simulink library "Batteries"  (R2023b)
settings: Solver=VariableStepAuto  StartTime=0.0  StopTime=10.0  RelTol=1e-3
undefined symbols (not defined in the file or in its folder): battery_builder_rtmsupport, gcbh
libraries: Batteries_lib x8
(part 1 of 4)
settings Model: Creator=maxju  LastModifiedBy=maxju

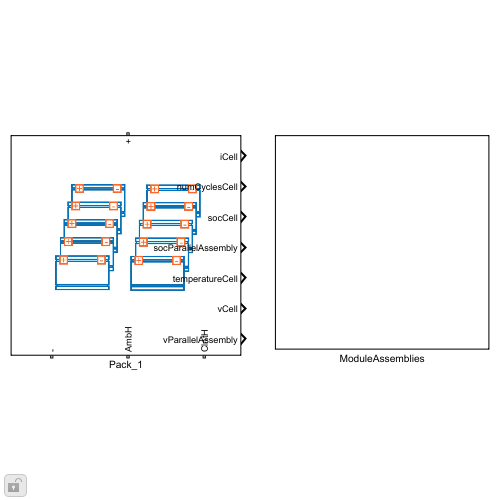
[thumbnail: Simulink's stored preview of the top-level diagram]
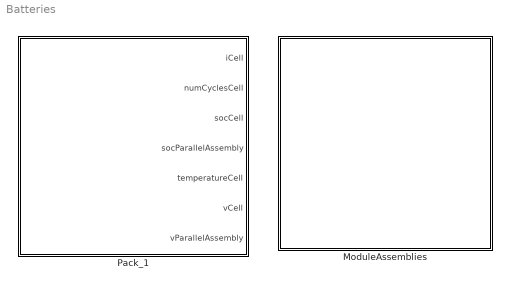
== system Batteries ==
  ModuleAssemblies : Subsystem
  Pack_1 : Subsystem  LoadFcn=battery_builder_rtmsupport('loadfcn',gcbh);
      settings: CopyFcn=battery_builder_rtmsupport('copyfcn',gcbh);  PreCopyFcn=battery_builder_rtmsupport('precopyfcn',gcbh);  PreDeleteFcn=battery_builder_rtmsupport('predeletefcn',gcbh);  PortSchema="{\"entries\":[{\"content\":{\"sides\":[{\"content\":{\"connectorIds\":[\"LConn1\"]},\"type\":\"ConnectorPlacement.EquallySpacedRectSide\",\"uuid\":\"3208743a-a519-41a1-8ebe-6eed9670d19c\"},{\"content\":{\"connectorIds\":[\"RConn1\",\"RConn2\",\"RConn3\"],\"side\":\"RIGHT\"},\"type\":\"ConnectorPlacement.EquallySpacedRectSide\",\"uuid\":\"e7c9afcf-26e4-4003-a175-67ec4307a0b6\"},{\"content\":{\"side\":\"TOP\"},\"type\":\"ConnectorPlacement.EquallySpacedRectSide\",\"uuid\":\"e113849d-7e09-4ac7-ac0d-e10ce5f1c420\"},{\"content\":{\"connectorIds\":[\"Out1\",\"Out2\",\"Out3\",\"Out4\",\"Out5\",\"Out6\",\"Out7\"],\"side\":\"BOTTOM\"},\"type\":\"ConnectorPlacement.EquallySpacedRectSide\",\"uuid\":\"7e3d0ba5-349a-464e-b9e7-0ee2ee84a6c1\"}]},\"type\":\"ConnectorPlacement.EquallySpacedConnector\",\"uuid\":\"9e673d86-8bc3-4af2-b5cc-e8b6c563b87a\"}],\"packageUris\":[\"http://schema.mathworks.com/mf0/Connector/R2020b\"],\"version\":\"1.0\"}"
      mask Display: image('$imagefile')

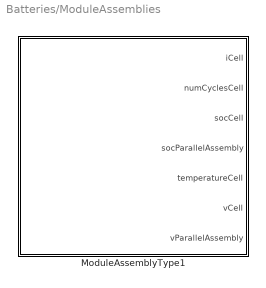
== system Batteries/ModuleAssemblies ==
  ModuleAssemblyType1 : Subsystem  LoadFcn=battery_builder_rtmsupport('loadfcn',gcbh);
      settings: CopyFcn=battery_builder_rtmsupport('copyfcn',gcbh);  PreCopyFcn=battery_builder_rtmsupport('precopyfcn',gcbh);  PreDeleteFcn=battery_builder_rtmsupport('predeletefcn',gcbh);  PortSchema="{\"entries\":[{\"content\":{\"sides\":[{\"content\":{\"connectorIds\":[\"LConn1\"]},\"type\":\"ConnectorPlacement.EquallySpacedRectSide\",\"uuid\":\"3208743a-a519-41a1-8ebe-6eed9670d19c\"},{\"content\":{\"connectorIds\":[\"RConn1\",\"RConn2\",\"RConn3\"],\"side\":\"RIGHT\"},\"type\":\"ConnectorPlacement.EquallySpacedRectSide\",\"uuid\":\"e7c9afcf-26e4-4003-a175-67ec4307a0b6\"},{\"content\":{\"side\":\"TOP\"},\"type\":\"ConnectorPlacement.EquallySpacedRectSide\",\"uuid\":\"e113849d-7e09-4ac7-ac0d-e10ce5f1c420\"},{\"content\":{\"connectorIds\":[\"Out1\",\"Out2\",\"Out3\",\"Out4\",\"Out5\",\"Out6\",\"Out7\"],\"side\":\"BOTTOM\"},\"type\":\"ConnectorPlacement.EquallySpacedRectSide\",\"uuid\":\"c73d48af-17c4-4fef-bb81-c5ffd3e9339e\"}]},\"type\":\"ConnectorPlacement.EquallySpacedConnector\",\"uuid\":\"9e673d86-8bc3-4af2-b5cc-e8b6c563b87a\"}],\"packageUris\":[\"http://schema.mathworks.com/mf0/Connector/R2020b\"],\"version\":\"1.0\"}"
      mask Display: image('$imagefile')

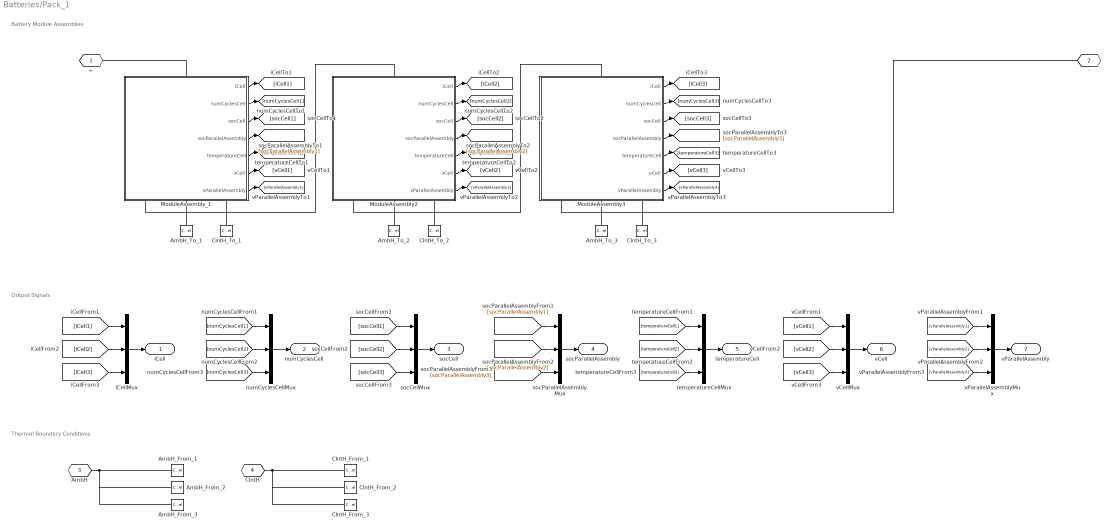
== system Batteries/Pack_1 ==
  note: Battery Module Assemblies
  note: Output Signals
  note: Thermal Boundary Conditions
  AmbH_From_1 : ConnectionLabel  Label=ambH_1
  AmbH_From_2 : ConnectionLabel  Label=ambH_2
  AmbH_From_3 : ConnectionLabel  Label=ambH_3
  AmbH_To_1 : ConnectionLabel  Label=ambH_1
  AmbH_To_2 : ConnectionLabel  Label=ambH_2
  AmbH_To_3 : ConnectionLabel  Label=ambH_3
  ClntH_From_1 : ConnectionLabel  Label=clntH_1
  ClntH_From_2 : ConnectionLabel  Label=clntH_2
  ClntH_From_3 : ConnectionLabel  Label=clntH_3
  ClntH_To_1 : ConnectionLabel  Label=clntH_1
  ClntH_To_2 : ConnectionLabel  Label=clntH_2
  ClntH_To_3 : ConnectionLabel  Label=clntH_3
  ModuleAssembly2 : Subsystem  LoadFcn=battery_builder_rtmsupport('loadfcn',gcbh);
      settings: CopyFcn=battery_builder_rtmsupport('copyfcn',gcbh);  PreCopyFcn=battery_builder_rtmsupport('precopyfcn',gcbh);  PreDeleteFcn=battery_builder_rtmsupport('predeletefcn',gcbh);  PortSchema="{\"entries\":[{\"content\":{\"sides\":[{\"content\":{\"connectorIds\":[\"LConn1\"]},\"type\":\"ConnectorPlacement.EquallySpacedRectSide\",\"uuid\":\"3208743a-a519-41a1-8ebe-6eed9670d19c\"},{\"content\":{\"connectorIds\":[\"RConn1\",\"RConn2\",\"RConn3\"],\"side\":\"RIGHT\"},\"type\":\"ConnectorPlacement.EquallySpacedRectSide\",\"uuid\":\"e7c9afcf-26e4-4003-a175-67ec4307a0b6\"},{\"content\":{\"side\":\"TOP\"},\"type\":\"ConnectorPlacement.EquallySpacedRectSide\",\"uuid\":\"e113849d-7e09-4ac7-ac0d-e10ce5f1c420\"},{\"content\":{\"connectorIds\":[\"Out1\",\"Out2\",\"Out3\",\"Out4\",\"Out5\",\"Out6\",\"Out7\"],\"side\":\"BOTTOM\"},\"type\":\"ConnectorPlacement.EquallySpacedRectSide\",\"uuid\":\"c73d48af-17c4-4fef-bb81-c5ffd3e9339e\"}]},\"type\":\"ConnectorPlacement.EquallySpacedConnector\",\"uuid\":\"9e673d86-8bc3-4af2-b5cc-e8b6c563b87a\"}],\"packageUris\":[\"http://schema.mathworks.com/mf0/Connector/R2020b\"],\"version\":\"1.0\"}"
      mask Display: image('$imagefile')
  ModuleAssembly3 : Subsystem  LoadFcn=battery_builder_rtmsupport('loadfcn',gcbh);
      settings: CopyFcn=battery_builder_rtmsupport('copyfcn',gcbh);  PreCopyFcn=battery_builder_rtmsupport('precopyfcn',gcbh);  PreDeleteFcn=battery_builder_rtmsupport('predeletefcn',gcbh);  PortSchema="{\"entries\":[{\"content\":{\"sides\":[{\"content\":{\"connectorIds\":[\"LConn1\"]},\"type\":\"ConnectorPlacement.EquallySpacedRectSide\",\"uuid\":\"3208743a-a519-41a1-8ebe-6eed9670d19c\"},{\"content\":{\"connectorIds\":[\"RConn1\",\"RConn2\",\"RConn3\"],\"side\":\"RIGHT\"},\"type\":\"ConnectorPlacement.EquallySpacedRectSide\",\"uuid\":\"e7c9afcf-26e4-4003-a175-67ec4307a0b6\"},{\"content\":{\"side\":\"TOP\"},\"type\":\"ConnectorPlacement.EquallySpacedRectSide\",\"uuid\":\"e113849d-7e09-4ac7-ac0d-e10ce5f1c420\"},{\"content\":{\"connectorIds\":[\"Out1\",\"Out2\",\"Out3\",\"Out4\",\"Out5\",\"Out6\",\"Out7\"],\"side\":\"BOTTOM\"},\"type\":\"ConnectorPlacement.EquallySpacedRectSide\",\"uuid\":\"c73d48af-17c4-4fef-bb81-c5ffd3e9339e\"}]},\"type\":\"ConnectorPlacement.EquallySpacedConnector\",\"uuid\":\"9e673d86-8bc3-4af2-b5cc-e8b6c563b87a\"}],\"packageUris\":[\"http://schema.mathworks.com/mf0/Connector/R2020b\"],\"version\":\"1.0\"}"
      mask Display: image('$imagefile')
  ModuleAssembly_1 : Subsystem  LoadFcn=battery_builder_rtmsupport('loadfcn',gcbh);
      settings: CopyFcn=battery_builder_rtmsupport('copyfcn',gcbh);  PreCopyFcn=battery_builder_rtmsupport('precopyfcn',gcbh);  PreDeleteFcn=battery_builder_rtmsupport('predeletefcn',gcbh);  PortSchema="{\"entries\":[{\"content\":{\"sides\":[{\"content\":{\"connectorIds\":[\"LConn1\"]},\"type\":\"ConnectorPlacement.EquallySpacedRectSide\",\"uuid\":\"3208743a-a519-41a1-8ebe-6eed9670d19c\"},{\"content\":{\"connectorIds\":[\"RConn1\",\"RConn2\",\"RConn3\"],\"side\":\"RIGHT\"},\"type\":\"ConnectorPlacement.EquallySpacedRectSide\",\"uuid\":\"e7c9afcf-26e4-4003-a175-67ec4307a0b6\"},{\"content\":{\"side\":\"TOP\"},\"type\":\"ConnectorPlacement.EquallySpacedRectSide\",\"uuid\":\"e113849d-7e09-4ac7-ac0d-e10ce5f1c420\"},{\"content\":{\"connectorIds\":[\"Out1\",\"Out2\",\"Out3\",\"Out4\",\"Out5\",\"Out6\",\"Out7\"],\"side\":\"BOTTOM\"},\"type\":\"ConnectorPlacement.EquallySpacedRectSide\",\"uuid\":\"c73d48af-17c4-4fef-bb81-c5ffd3e9339e\"}]},\"type\":\"ConnectorPlacement.EquallySpacedConnector\",\"uuid\":\"9e673d86-8bc3-4af2-b5cc-e8b6c563b87a\"}],\"packageUris\":[\"http://schema.mathworks.com/mf0/Connector/R2020b\"],\"version\":\"1.0\"}"
      mask Display: image('$imagefile')
  iCellMux : Mux  Inputs=3
  numCyclesCellMux : Mux  Inputs=3
  socCellMux : Mux  Inputs=3
  socParallelAssemblyMux : Mux  Inputs=3
  temperatureCellMux : Mux  Inputs=3
  vCellMux : Mux  Inputs=3
  vParallelAssemblyMux : Mux  Inputs=3
  + : PMIOPort  Side=Left
  - : PMIOPort  Port=2  Side=Right
  AmbH : PMIOPort  Port=3  Side=Right  ConnectionType=Connection: foundation.thermal.thermal
  ClntH : PMIOPort  Port=4  Side=Right  ConnectionType=Connection: foundation.thermal.thermal
  iCell : Outport
  numCyclesCell : Outport  Port=2
  socCell : Outport  Port=3
  socParallelAssembly : Outport  Port=4
  temperatureCell : Outport  Port=5
  vCell : Outport  Port=6
  vParallelAssembly : Outport  Port=7
  wires:
  ModuleAssembly_1/1(iCell) -> [iCell1]
  iCellMux/1 -> iCell/1
  [iCell1] -> iCellMux/1
  ModuleAssembly_1/2(numCyclesCell) -> [numCyclesCell1]
  numCyclesCellMux/1 -> numCyclesCell/1
  [numCyclesCell1] -> numCyclesCellMux/1
  ModuleAssembly_1/3(socCell) -> [socCell1]
  socCellMux/1 -> socCell/1
  [socCell1] -> socCellMux/1
  ModuleAssembly_1/4(socParallelAssembly) -> [socParallelAssembly1]
  socParallelAssemblyMux/1 -> socParallelAssembly/1
  [socParallelAssembly1] -> socParallelAssemblyMux/1
  ModuleAssembly_1/5(temperatureCell) -> [temperatureCell1]
  temperatureCellMux/1 -> temperatureCell/1
  [temperatureCell1] -> temperatureCellMux/1
  ModuleAssembly_1/6(vCell) -> [vCell1]
  vCellMux/1 -> vCell/1
  [vCell1] -> vCellMux/1
  ModuleAssembly_1/7(vParallelAssembly) -> [vParallelAssembly1]
  vParallelAssemblyMux/1 -> vParallelAssembly/1
  [vParallelAssembly1] -> vParallelAssemblyMux/1
  ModuleAssembly2/1(iCell) -> [iCell2]
  [iCell2] -> iCellMux/2
  ModuleAssembly2/2(numCyclesCell) -> [numCyclesCell2]
  [numCyclesCell2] -> numCyclesCellMux/2
  ModuleAssembly2/3(socCell) -> [socCell2]
  [socCell2] -> socCellMux/2
  ModuleAssembly2/4(socParallelAssembly) -> [socParallelAssembly2]
  [socParallelAssembly2] -> socParallelAssemblyMux/2
  ModuleAssembly2/5(temperatureCell) -> [temperatureCell2]
  [temperatureCell2] -> temperatureCellMux/2
  ModuleAssembly2/6(vCell) -> [vCell2]
  [vCell2] -> vCellMux/2
  ModuleAssembly2/7(vParallelAssembly) -> [vParallelAssembly2]
  [vParallelAssembly2] -> vParallelAssemblyMux/2
  ModuleAssembly3/1(iCell) -> [iCell3]
  [iCell3] -> iCellMux/3
  ModuleAssembly3/2(numCyclesCell) -> [numCyclesCell3]
  [numCyclesCell3] -> numCyclesCellMux/3
  ModuleAssembly3/3(socCell) -> [socCell3]
  [socCell3] -> socCellMux/3
  ModuleAssembly3/4(socParallelAssembly) -> [socParallelAssembly3]
  [socParallelAssembly3] -> socParallelAssemblyMux/3
  ModuleAssembly3/5(temperatureCell) -> [temperatureCell3]
  [temperatureCell3] -> temperatureCellMux/3
  ModuleAssembly3/6(vCell) -> [vCell3]
  [vCell3] -> vCellMux/3
  ModuleAssembly3/7(vParallelAssembly) -> [vParallelAssembly3]
  [vParallelAssembly3] -> vParallelAssemblyMux/3
  connections:
  ModuleAssembly2/LConn1 -- ModuleAssembly_1/RConn1
  ModuleAssembly3/LConn1 -- ModuleAssembly2/RConn1
  ModuleAssembly_1/LConn1 -- +/RConn1
  ModuleAssembly3/RConn1 -- -/RConn1
  AmbH_To_1/LConn1 -- ModuleAssembly_1/RConn2
  AmbH_From_1/LConn1 -- AmbH_From_2/LConn1 -- AmbH/RConn1 -- AmbH_From_3/LConn1
  AmbH_To_2/LConn1 -- ModuleAssembly2/RConn2
  AmbH_To_3/LConn1 -- ModuleAssembly3/RConn2
  ClntH_To_1/LConn1 -- ModuleAssembly_1/RConn3
  ClntH_From_1/LConn1 -- ClntH_From_2/LConn1 -- ClntH/RConn1 -- ClntH_From_3/LConn1
  ClntH_To_2/LConn1 -- ModuleAssembly2/RConn3
  ClntH_To_3/LConn1 -- ModuleAssembly3/RConn3

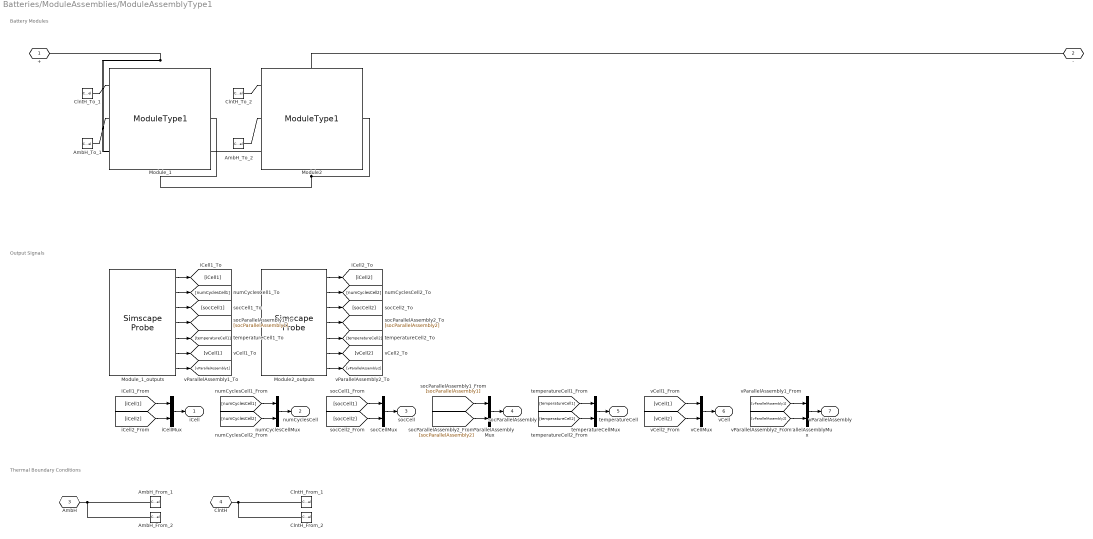
== system Batteries/ModuleAssemblies/ModuleAssemblyType1 ==
  note: Battery Modules
  note: Output Signals
  note: Thermal Boundary Conditions
  AmbH_From_1 : ConnectionLabel  Label=ambH_1
  AmbH_From_2 : ConnectionLabel  Label=ambH_2
  AmbH_To_1 : ConnectionLabel  Label=ambH_1
  AmbH_To_2 : ConnectionLabel  Label=ambH_2
  ClntH_From_1 : ConnectionLabel  Label=clntH_1
  ClntH_From_2 : ConnectionLabel  Label=clntH_2
  ClntH_To_1 : ConnectionLabel  Label=clntH_1
  ClntH_To_2 : ConnectionLabel  Label=clntH_2
  Module2 : Batteries_lib/Modules/ModuleType1  SOC_vecCell=[0, .01, .02, .03, .04, .05, .06, .07, .08, .09, .1, .11, .12, .13, .14, .15, .16, .17, .18, .19, .2, .21, .22, .23, .24, .25, .26, .27, .28, .29, .3, .31, .32, .33, .34, .35, .36, .37, .38, .39, .4, .41, .42, .43, .44, .45, .46, .47, .48, .49, .5, .51, .52, .53, .54, .55, .56, .57, .58, .59, .6, .61, .62, .63, .64, .65, .66, .67, .68, .69, .7, .71, .72, .73, .74, .75, .76, .77, .78, .79, .8, .81, .82, .83, .84, .85, .86, .87, .88, .89, .9, .91, .92, .93, .94, .95, .96, .97, .98, .99, 1]  T_vecCell=[-10, 0, 25, 40, 60] degC  V0_matCell=[2.90003, 2.90003, 2.90003, 2.90003, 2.90003; 2.94341, 2.94341, 2.94341, 2.94341, 2.94341; 2.98679, 2.98679, 2.98679, 2.98679, 2.98679; 3.04987, 3.04987, 3.04987, 3.04987, 3.04987; 3.09433, 3.09433, 3.09433, 3.09433, 3.09433; 3.12791, 3.12791, 3.12791, 3.12791, 3.12791; 3.16031, 3.16031, 3.16031, 3.16031, 3.16031; 3.20369, 3.20369, 3.20369, 3.20369, 3.20369; 3.23862, 3.23862, 3.23862, 3.23862, 3.23862; 3.26689, 3.26689, 3.26689, 3.26689, 3.26689; 3.29115, 3.29115, 3.29115, 3.29115, 3.29115; 3.31383, 3.31383, 3.31383, 3.31383, 3.31383; 3.33202, 3.33202, 3.33202, 3.33202, 3.33202; 3.35112, 3.35112, 3.35112, 3.35112, 3.35112; 3.36833, 3.36833, 3.36833, 3.36833, 3.36833; 3.38413, 3.38413, 3.38413, 3.38413, 3.38413; 3.39973, 3.39973, 3.39973, 3.39973, 3.39973; 3.41137, 3.41137, 3.41137, 3.41137, 3.41137; 3.42149, 3.42149, 3.42149, 3.42149, 3.42149; 3.43136, 3.43136, 3.43136, 3.43136, 3.43136; 3.44073, 3.44073, 3.44073, 3.44073, 3.44073; 3.45027, 3.45027, 3.45027, 3.45027, 3.45027; 3.46068, 3.46068, 3.46068, 3.46068, 3.46068; 3.47113, 3.47113, 3.47113, 3.47113, 3.47113; 3.47814, 3.47814, 3.47814, 3.47814, 3.47814; 3.48494, 3.48494, 3.48494, 3.48494, 3.48494; 3.49199, 3.49199, 3.49199, 3.49199, 3.49199; 3.49905, 3.49905, 3.49905, 3.49905, 3.49905; 3.50562, 3.50562, 3.50562, 3.50562, 3.50562; 3.51187, 3.51187, 3.51187, 3.51187, 3.51187; 3.51861, 3.51861, 3.51861, 3.51861, 3.51861; 3.52535, 3.52535, 3.52535, 3.52535, 3.52535; 3.53209, 3.53209, 3.53209, 3.53209, 3.53209; 3.53818, 3.53818, 3.53818, 3.53818, 3.53818; 3.54353, 3.54353, 3.54353, 3.54353, 3.54353; 3.54849, 3.54849, 3.54849, 3.54849, 3.54849; 3.55353, 3.55353, 3.55353, 3.55353, 3.55353; 3.55855, 3.55855, 3.55855, 3.55855, 3.55855; 3.56357, 3.56357, 3.56357, 3.56357, 3.56357; 3.56831, 3.56831, 3.56831, 3.56831, 3.56831; 3.57308, 3.57308, 3.57308, 3.57308, 3.57308; 3.57787, 3.57787, 3.57787, 3.57787, 3.57787; 3.58264, 3.58264, 3.58264, 3.58264, 3.58264; 3.58755, 3.58755, 3.58755, 3.58755, 3.58755; 3.5925, 3.5925, 3.5925, 3.5925, 3.5925; 3.5985, 3.5985, 3.5985, 3.5985, 3.5985; 3.60496, 3.60496, 3.60496, 3.60496, 3.60496; 3.61149, 3.61149, 3.61149, 3.61149, 3.61149; 3.61805, 3.61805, 3.61805, 3.61805, 3.61805; 3.6246, 3.6246, 3.6246, 3.6246, 3.6246; 3.63116, 3.63116, 3.63116, 3.63116, 3.63116; 3.63855, 3.63855, 3.63855, 3.63855, 3.63855; 3.64609, 3.64609, 3.64609, 3.64609, 3.64609; 3.65336, 3.65336, 3.65336, 3.65336, 3.65336; 3.66064, 3.66064, 3.66064, 3.66064, 3.66064; 3.66791, 3.66791, 3.66791, 3.66791, 3.66791; 3.67613, 3.67613, 3.67613, 3.67613, 3.67613; 3.68522, 3.68522, 3.68522, 3.68522, 3.68522; 3.69443, 3.69443, 3.69443, 3.69443, 3.69443; 3.70367, 3.70367, 3.70367, 3.70367, 3.70367; 3.713, 3.713, 3.713, 3.713, 3.713; 3.72241, 3.72241, 3.72241, 3.72241, 3.72241; 3.73154, 3.73154, 3.73154, 3.73154, 3.73154; 3.74037, 3.74037, 3.74037, 3.74037, 3.74037; 3.7492, 3.7492, 3.7492, 3.7492, 3.7492; 3.75786, 3.75786, 3.75786, 3.75786, 3.75786; 3.76617, 3.76617, 3.76617, 3.76617, 3.76617; 3.77556, 3.77556, 3.77556, 3.77556, 3.77556; 3.78485, 3.78485, 3.78485, 3.78485, 3.78485; 3.79413, 3.79413, 3.79413, 3.79413, 3.79413; 3.8034, 3.8034, 3.8034, 3.8034, 3.8034; 3.81149, 3.81149, 3.81149, 3.81149, 3.81149; 3.81977, 3.81977, 3.81977, 3.81977, 3.81977; 3.82804, 3.82804, 3.82804, 3.82804, 3.82804; 3.83631, 3.83631, 3.83631, 3.83631, 3.83631; 3.84472, 3.84472, 3.84472, 3.84472, 3.84472; 3.85317, 3.85317, 3.85317, 3.85317, 3.85317; 3.86155, 3.86155, 3.86155, 3.86155, 3.86155; 3.86993, 3.86993, 3.86993, 3.86993, 3.86993; 3.87831, 3.87831, 3.87831, 3.87831, 3.87831; 3.88686, 3.88686, 3.88686, 3.88686, 3.88686; 3.89534, 3.89534, 3.89534, 3.89534, 3.89534; 3.90461, 3.90461, 3.90461, 3.90461, 3.90461; 3.91454, 3.91454, 3.91454, 3.91454, 3.91454; 3.92565, 3.92565, 3.92565, 3.92565, 3.92565; 3.93721, 3.93721, 3.93721, 3.93721, 3.93721; 3.94924, 3.94924, 3.94924, 3.94924, 3.94924; 3.96155, 3.96155, 3.96155, 3.96155, 3.96155; 3.97383, 3.97383, 3.97383, 3.97383, 3.97383; 3.98598, 3.98598, 3.98598, ...(+512 chars)] V  V_rangeCell=[2.25, Inf] V  R0_matCell=[.54124, .47218, .1741, .16472, .13072; .60048, .51942, .15823, .09801, .03241; .57827, .49613, .14313, .06257, .00499; .55606, .47283, .13285, .0492, .00058; .53384, .44953, .12044, .03857, .00058; .51163, .42624, .10641, .0337, .00058; .48942, .40294, .09605, .03258, .00058; .46721, .37965, .09162, .03508, .0103; .44499, .35635, .08758, .0376, .01722; .42278, .33305, .08349, .04115, .02235; .40057, .30976, .08021, .04338, .0273; .37836, .28646, .07738, .04509, .03173; .35615, .26317, .07487, .04551, .03469; .33393, .24021, .07338, .04781, .03783; .31172, .21801, .07189, .04948, .04012; .28951, .203, .07117, .05069, .04195; .26873, .19013, .0704, .05182, .04371; .24946, .17834, .06898, .05166, .04417; .23189, .16793, .06755, .05143, .04397; .21926, .15878, .06631, .0513, .04362; .2084, .15119, .06509, .05101, .04311; .19882, .14534, .06388, .05077, .04265; .19282, .14029, .06326, .05091, .04272; .18782, .13679, .06281, .05124, .04325; .18252, .13215, .06182, .05043, .04264; .17725, .12766, .06095, .04955, .04196; .173, .125, .06025, .04876, .04137; .16875, .12234, .05955, .04802, .04078; .16459, .11952, .05877, .04782, .04033; .16124, .11704, .05807, .04752, .03993; .15805, .11494, .05761, .04737, .03969; .15486, .11285, .05714, .04723, .03945; .15212, .11075, .05668, .04709, .03921; .15022, .10906, .05611, .04673, .03878; .14807, .10773, .05546, .04612, .03867; .14579, .10628, .0549, .04546, .03843; .14353, .10484, .05439, .04485, .03821; .14127, .10351, .05388, .04423, .03799; .13957, .10228, .05337, .04361, .03777; .13785, .10097, .0528, .0429, .03746; .13614, .09966, .05223, .0422, .0367; .13443, .09836, .05165, .04151, .03572; .13272, .09711, .05106, .04111, .03474; .13096, .09591, .05046, .04079, .03381; .12918, .09471, .04986, .04049, .03288; .12775, .09387, .04945, .04053, .03231; .12648, .09317, .04913, .04073, .03189; .12522, .09249, .04883, .04095, .03151; .12398, .09181, .04854, .04066, .03136; .12296, .09112, .04826, .04006, .03121; .12207, .09044, .04797, .03947, .03106; .12147, .09003, .04782, .03916, .03119; .12091, .08967, .04765, .03889, .03136; .12027, .08886, .0473, .03854, .03145; .11955, .08797, .04695, .03818, .03154; .11836, .08708, .04661, .03764, .03136; .11749, .08651, .04638, .03733, .03126; .1169, .08628, .0463, .03731, .03144; .11636, .0866, .04625, .03733, .03167; .11679, .08693, .04621, .03736, .0319; .11639, .08729, .04624, .03741, .03216; .11602, .08748, .04628, .0375, .03245; .11556, .08747, .04628, .03749, .03262; .115, .08737, .04623, .03738, .03268; .11444, .08726, .04617, .03728, .03275; .11413, .08683, .04599, .03714, .03276; .11369, .08629, .04573, .03712, .03265; .11362, .0861, .0457, .03746, .03289; .11351, .08597, .04568, .03777, .03289; .1134, .08596, .04565, .03807, .03285; .11329, .08593, .04563, .03837, .0328; .11297, .08552, .04535, .03804, .03236; .1131, .0855, .0451, .03769, .03198; .11323, .08564, .04486, .03733, .0316; .11336, .08578, .04461, .03698, .03122; .11354, .08596, .04446, .03667, .03091; .11376, .08614, .04435, .03629, .0306; .11421, .08628, .04423, .03577, .03027; .11467, .08641, .04411, .03525, .02995; .11513, .08655, .044, .03473, .02961; .11565, .08679, .04372, .03426, .02933; .11614, .08704, .04339, .03378, .02903; .11689, .08756, .04323, .03353, .02899; .11825, .08829, .0432, .03328, .02916; .12033, .08941, .04344, .03342, .02973; .12256, .09067, .04374, .03371, .0301; .12495, .09191, .0441, .03415, .02981; .12743, .09323, .04452, .03468, .0296; .13108, .09454, .04494, .03488, .02939; .13509, .09581, .0454, .03488, .02914; .13924, .09835, .04594, .03502, .02907; .14357, .1012, .0463, .03517, .02937; .14857, .10399, .04649, .03528, .02963; .15358, .10679, .04668, .03541, .02989; .15894, .10894, .04629, .035, .02961; .16451, .11073, .04541, .03434, .02892; .17255, .11235, .04438, .03375, .02804; .17994, .11383, .04326, .03305, .02704; .18615, .11422, .04154, .03252, .02601; .19123, .11362, .03869, .03189, .02484; .17773, .09538, .03326, .0315, .0239] Ohm  AHCell=3.153 A*hr  extrapolation_optionCell=simscape.enum.extrapolation.nearest  thermal_massCell=44.55 J/K  CoolantResistance=1.2 K/W  AmbientResistance=25 K/W  P=3  S=3  iCell_specify=off  iCell_priority=None  iCell=0 A  iCell_nominal_specify=off  iCell_nominal_unit=A  iCell_nominal_value=1  vCell_specify=off  vCell_priority=None  vCell=0 V  vCell_nominal_specify=off  vCell_nominal_unit=V  vCell_nominal_value=1  socCell_specify=off  socCell_priority=High  socCell=1  socCell_nominal_specify=off  socCell_nominal_unit=1  socCell_nominal_value=1  numCyclesCell_specify=off  numCyclesCell_priority=High  numCyclesCell=0  numCyclesCell_nominal_specify=off  numCyclesCell_nominal_unit=1  numCyclesCell_nominal_value=1  temperatureCell_specify=off  temperatureCell_priority=High  temperatureCell=298.15 K  temperatureCell_nominal_specify=off  temperatureCell_nominal_unit=K  temperatureCell_nominal_value=1  vParallelAssembly_specify=off  vParallelAssembly_priority=None  vParallelAssembly=repmat(0, 3, 1) V  vParallelAssembly_nominal_specify=off  vParallelAssembly_nominal_unit=V  vParallelAssembly_nominal_value=1  socParallelAssembly_specify=off  socParallelAssembly_priority=None  socParallelAssembly=repmat(1, 3, 1)  socParallelAssembly_nominal_specify=off  socParallelAssembly_nominal_unit=1  socParallelAssembly_nominal_value=1
      settings: InternalSimscapePortConfiguration="{\"Bottom\":[{\"id\":\"n\",\"label\":\"-\",\"type\":\"foundation.electrical.electrical\"}],\"Left\":[{\"id\":\"ClntH\",\"label\":\"ClntH\",\"type\":\"foundation.thermal.thermal\"},{\"id\":\"AmbH\",\"label\":\"AmbH\",\"type\":\"foundation.thermal.thermal\"}],\"Right\":[],\"Top\":[{\"id\":\"p\",\"label\":\"+\",\"type\":\"foundation.electrical.electrical\"}]}"
  Module2_outputs : SimscapeProbe  BoundBlock=4  Variables={iCell, numCyclesCell, socCell, socParallelAssembly, temperatureCell, vCell, vParallelAssembly}
  Module_1 : Batteries_lib/Modules/ModuleType1  SOC_vecCell=[0, .01, .02, .03, .04, .05, .06, .07, .08, .09, .1, .11, .12, .13, .14, .15, .16, .17, .18, .19, .2, .21, .22, .23, .24, .25, .26, .27, .28, .29, .3, .31, .32, .33, .34, .35, .36, .37, .38, .39, .4, .41, .42, .43, .44, .45, .46, .47, .48, .49, .5, .51, .52, .53, .54, .55, .56, .57, .58, .59, .6, .61, .62, .63, .64, .65, .66, .67, .68, .69, .7, .71, .72, .73, .74, .75, .76, .77, .78, .79, .8, .81, .82, .83, .84, .85, .86, .87, .88, .89, .9, .91, .92, .93, .94, .95, .96, .97, .98, .99, 1]  T_vecCell=[-10, 0, 25, 40, 60] degC  V0_matCell=[2.90003, 2.90003, 2.90003, 2.90003, 2.90003; 2.94341, 2.94341, 2.94341, 2.94341, 2.94341; 2.98679, 2.98679, 2.98679, 2.98679, 2.98679; 3.04987, 3.04987, 3.04987, 3.04987, 3.04987; 3.09433, 3.09433, 3.09433, 3.09433, 3.09433; 3.12791, 3.12791, 3.12791, 3.12791, 3.12791; 3.16031, 3.16031, 3.16031, 3.16031, 3.16031; 3.20369, 3.20369, 3.20369, 3.20369, 3.20369; 3.23862, 3.23862, 3.23862, 3.23862, 3.23862; 3.26689, 3.26689, 3.26689, 3.26689, 3.26689; 3.29115, 3.29115, 3.29115, 3.29115, 3.29115; 3.31383, 3.31383, 3.31383, 3.31383, 3.31383; 3.33202, 3.33202, 3.33202, 3.33202, 3.33202; 3.35112, 3.35112, 3.35112, 3.35112, 3.35112; 3.36833, 3.36833, 3.36833, 3.36833, 3.36833; 3.38413, 3.38413, 3.38413, 3.38413, 3.38413; 3.39973, 3.39973, 3.39973, 3.39973, 3.39973; 3.41137, 3.41137, 3.41137, 3.41137, 3.41137; 3.42149, 3.42149, 3.42149, 3.42149, 3.42149; 3.43136, 3.43136, 3.43136, 3.43136, 3.43136; 3.44073, 3.44073, 3.44073, 3.44073, 3.44073; 3.45027, 3.45027, 3.45027, 3.45027, 3.45027; 3.46068, 3.46068, 3.46068, 3.46068, 3.46068; 3.47113, 3.47113, 3.47113, 3.47113, 3.47113; 3.47814, 3.47814, 3.47814, 3.47814, 3.47814; 3.48494, 3.48494, 3.48494, 3.48494, 3.48494; 3.49199, 3.49199, 3.49199, 3.49199, 3.49199; 3.49905, 3.49905, 3.49905, 3.49905, 3.49905; 3.50562, 3.50562, 3.50562, 3.50562, 3.50562; 3.51187, 3.51187, 3.51187, 3.51187, 3.51187; 3.51861, 3.51861, 3.51861, 3.51861, 3.51861; 3.52535, 3.52535, 3.52535, 3.52535, 3.52535; 3.53209, 3.53209, 3.53209, 3.53209, 3.53209; 3.53818, 3.53818, 3.53818, 3.53818, 3.53818; 3.54353, 3.54353, 3.54353, 3.54353, 3.54353; 3.54849, 3.54849, 3.54849, 3.54849, 3.54849; 3.55353, 3.55353, 3.55353, 3.55353, 3.55353; 3.55855, 3.55855, 3.55855, 3.55855, 3.55855; 3.56357, 3.56357, 3.56357, 3.56357, 3.56357; 3.56831, 3.56831, 3.56831, 3.56831, 3.56831; 3.57308, 3.57308, 3.57308, 3.57308, 3.57308; 3.57787, 3.57787, 3.57787, 3.57787, 3.57787; 3.58264, 3.58264, 3.58264, 3.58264, 3.58264; 3.58755, 3.58755, 3.58755, 3.58755, 3.58755; 3.5925, 3.5925, 3.5925, 3.5925, 3.5925; 3.5985, 3.5985, 3.5985, 3.5985, 3.5985; 3.60496, 3.60496, 3.60496, 3.60496, 3.60496; 3.61149, 3.61149, 3.61149, 3.61149, 3.61149; 3.61805, 3.61805, 3.61805, 3.61805, 3.61805; 3.6246, 3.6246, 3.6246, 3.6246, 3.6246; 3.63116, 3.63116, 3.63116, 3.63116, 3.63116; 3.63855, 3.63855, 3.63855, 3.63855, 3.63855; 3.64609, 3.64609, 3.64609, 3.64609, 3.64609; 3.65336, 3.65336, 3.65336, 3.65336, 3.65336; 3.66064, 3.66064, 3.66064, 3.66064, 3.66064; 3.66791, 3.66791, 3.66791, 3.66791, 3.66791; 3.67613, 3.67613, 3.67613, 3.67613, 3.67613; 3.68522, 3.68522, 3.68522, 3.68522, 3.68522; 3.69443, 3.69443, 3.69443, 3.69443, 3.69443; 3.70367, 3.70367, 3.70367, 3.70367, 3.70367; 3.713, 3.713, 3.713, 3.713, 3.713; 3.72241, 3.72241, 3.72241, 3.72241, 3.72241; 3.73154, 3.73154, 3.73154, 3.73154, 3.73154; 3.74037, 3.74037, 3.74037, 3.74037, 3.74037; 3.7492, 3.7492, 3.7492, 3.7492, 3.7492; 3.75786, 3.75786, 3.75786, 3.75786, 3.75786; 3.76617, 3.76617, 3.76617, 3.76617, 3.76617; 3.77556, 3.77556, 3.77556, 3.77556, 3.77556; 3.78485, 3.78485, 3.78485, 3.78485, 3.78485; 3.79413, 3.79413, 3.79413, 3.79413, 3.79413; 3.8034, 3.8034, 3.8034, 3.8034, 3.8034; 3.81149, 3.81149, 3.81149, 3.81149, 3.81149; 3.81977, 3.81977, 3.81977, 3.81977, 3.81977; 3.82804, 3.82804, 3.82804, 3.82804, 3.82804; 3.83631, 3.83631, 3.83631, 3.83631, 3.83631; 3.84472, 3.84472, 3.84472, 3.84472, 3.84472; 3.85317, 3.85317, 3.85317, 3.85317, 3.85317; 3.86155, 3.86155, 3.86155, 3.86155, 3.86155; 3.86993, 3.86993, 3.86993, 3.86993, 3.86993; 3.87831, 3.87831, 3.87831, 3.87831, 3.87831; 3.88686, 3.88686, 3.88686, 3.88686, 3.88686; 3.89534, 3.89534, 3.89534, 3.89534, 3.89534; 3.90461, 3.90461, 3.90461, 3.90461, 3.90461; 3.91454, 3.91454, 3.91454, 3.91454, 3.91454; 3.92565, 3.92565, 3.92565, 3.92565, 3.92565; 3.93721, 3.93721, 3.93721, 3.93721, 3.93721; 3.94924, 3.94924, 3.94924, 3.94924, 3.94924; 3.96155, 3.96155, 3.96155, 3.96155, 3.96155; 3.97383, 3.97383, 3.97383, 3.97383, 3.97383; 3.98598, 3.98598, 3.98598, ...(+512 chars)] V  V_rangeCell=[2.25, Inf] V  R0_matCell=[.54124, .47218, .1741, .16472, .13072; .60048, .51942, .15823, .09801, .03241; .57827, .49613, .14313, .06257, .00499; .55606, .47283, .13285, .0492, .00058; .53384, .44953, .12044, .03857, .00058; .51163, .42624, .10641, .0337, .00058; .48942, .40294, .09605, .03258, .00058; .46721, .37965, .09162, .03508, .0103; .44499, .35635, .08758, .0376, .01722; .42278, .33305, .08349, .04115, .02235; .40057, .30976, .08021, .04338, .0273; .37836, .28646, .07738, .04509, .03173; .35615, .26317, .07487, .04551, .03469; .33393, .24021, .07338, .04781, .03783; .31172, .21801, .07189, .04948, .04012; .28951, .203, .07117, .05069, .04195; .26873, .19013, .0704, .05182, .04371; .24946, .17834, .06898, .05166, .04417; .23189, .16793, .06755, .05143, .04397; .21926, .15878, .06631, .0513, .04362; .2084, .15119, .06509, .05101, .04311; .19882, .14534, .06388, .05077, .04265; .19282, .14029, .06326, .05091, .04272; .18782, .13679, .06281, .05124, .04325; .18252, .13215, .06182, .05043, .04264; .17725, .12766, .06095, .04955, .04196; .173, .125, .06025, .04876, .04137; .16875, .12234, .05955, .04802, .04078; .16459, .11952, .05877, .04782, .04033; .16124, .11704, .05807, .04752, .03993; .15805, .11494, .05761, .04737, .03969; .15486, .11285, .05714, .04723, .03945; .15212, .11075, .05668, .04709, .03921; .15022, .10906, .05611, .04673, .03878; .14807, .10773, .05546, .04612, .03867; .14579, .10628, .0549, .04546, .03843; .14353, .10484, .05439, .04485, .03821; .14127, .10351, .05388, .04423, .03799; .13957, .10228, .05337, .04361, .03777; .13785, .10097, .0528, .0429, .03746; .13614, .09966, .05223, .0422, .0367; .13443, .09836, .05165, .04151, .03572; .13272, .09711, .05106, .04111, .03474; .13096, .09591, .05046, .04079, .03381; .12918, .09471, .04986, .04049, .03288; .12775, .09387, .04945, .04053, .03231; .12648, .09317, .04913, .04073, .03189; .12522, .09249, .04883, .04095, .03151; .12398, .09181, .04854, .04066, .03136; .12296, .09112, .04826, .04006, .03121; .12207, .09044, .04797, .03947, .03106; .12147, .09003, .04782, .03916, .03119; .12091, .08967, .04765, .03889, .03136; .12027, .08886, .0473, .03854, .03145; .11955, .08797, .04695, .03818, .03154; .11836, .08708, .04661, .03764, .03136; .11749, .08651, .04638, .03733, .03126; .1169, .08628, .0463, .03731, .03144; .11636, .0866, .04625, .03733, .03167; .11679, .08693, .04621, .03736, .0319; .11639, .08729, .04624, .03741, .03216; .11602, .08748, .04628, .0375, .03245; .11556, .08747, .04628, .03749, .03262; .115, .08737, .04623, .03738, .03268; .11444, .08726, .04617, .03728, .03275; .11413, .08683, .04599, .03714, .03276; .11369, .08629, .04573, .03712, .03265; .11362, .0861, .0457, .03746, .03289; .11351, .08597, .04568, .03777, .03289; .1134, .08596, .04565, .03807, .03285; .11329, .08593, .04563, .03837, .0328; .11297, .08552, .04535, .03804, .03236; .1131, .0855, .0451, .03769, .03198; .11323, .08564, .04486, .03733, .0316; .11336, .08578, .04461, .03698, .03122; .11354, .08596, .04446, .03667, .03091; .11376, .08614, .04435, .03629, .0306; .11421, .08628, .04423, .03577, .03027; .11467, .08641, .04411, .03525, .02995; .11513, .08655, .044, .03473, .02961; .11565, .08679, .04372, .03426, .02933; .11614, .08704, .04339, .03378, .02903; .11689, .08756, .04323, .03353, .02899; .11825, .08829, .0432, .03328, .02916; .12033, .08941, .04344, .03342, .02973; .12256, .09067, .04374, .03371, .0301; .12495, .09191, .0441, .03415, .02981; .12743, .09323, .04452, .03468, .0296; .13108, .09454, .04494, .03488, .02939; .13509, .09581, .0454, .03488, .02914; .13924, .09835, .04594, .03502, .02907; .14357, .1012, .0463, .03517, .02937; .14857, .10399, .04649, .03528, .02963; .15358, .10679, .04668, .03541, .02989; .15894, .10894, .04629, .035, .02961; .16451, .11073, .04541, .03434, .02892; .17255, .11235, .04438, .03375, .02804; .17994, .11383, .04326, .03305, .02704; .18615, .11422, .04154, .03252, .02601; .19123, .11362, .03869, .03189, .02484; .17773, .09538, .03326, .0315, .0239] Ohm  AHCell=3.153 A*hr  extrapolation_optionCell=simscape.enum.extrapolation.nearest  thermal_massCell=44.55 J/K  CoolantResistance=1.2 K/W  AmbientResistance=25 K/W  P=3  S=3  iCell_specify=off  iCell_priority=None  iCell=0 A  iCell_nominal_specify=off  iCell_nominal_unit=A  iCell_nominal_value=1  vCell_specify=off  vCell_priority=None  vCell=0 V  vCell_nominal_specify=off  vCell_nominal_unit=V  vCell_nominal_value=1  socCell_specify=off  socCell_priority=High  socCell=1  socCell_nominal_specify=off  socCell_nominal_unit=1  socCell_nominal_value=1  numCyclesCell_specify=off  numCyclesCell_priority=High  numCyclesCell=0  numCyclesCell_nominal_specify=off  numCyclesCell_nominal_unit=1  numCyclesCell_nominal_value=1  temperatureCell_specify=off  temperatureCell_priority=High  temperatureCell=298.15 K  temperatureCell_nominal_specify=off  temperatureCell_nominal_unit=K  temperatureCell_nominal_value=1  vParallelAssembly_specify=off  vParallelAssembly_priority=None  vParallelAssembly=repmat(0, 3, 1) V  vParallelAssembly_nominal_specify=off  vParallelAssembly_nominal_unit=V  vParallelAssembly_nominal_value=1  socParallelAssembly_specify=off  socParallelAssembly_priority=None  socParallelAssembly=repmat(1, 3, 1)  socParallelAssembly_nominal_specify=off  socParallelAssembly_nominal_unit=1  socParallelAssembly_nominal_value=1
      settings: InternalSimscapePortConfiguration="{\"Bottom\":[{\"id\":\"n\",\"label\":\"-\",\"type\":\"foundation.electrical.electrical\"}],\"Left\":[{\"id\":\"ClntH\",\"label\":\"ClntH\",\"type\":\"foundation.thermal.thermal\"},{\"id\":\"AmbH\",\"label\":\"AmbH\",\"type\":\"foundation.thermal.thermal\"}],\"Right\":[],\"Top\":[{\"id\":\"p\",\"label\":\"+\",\"type\":\"foundation.electrical.electrical\"}]}"
  Module_1_outputs : SimscapeProbe  BoundBlock=3  Variables={iCell, numCyclesCell, socCell, socParallelAssembly, temperatureCell, vCell, vParallelAssembly}
  iCellMux : Mux  Inputs=2
  numCyclesCellMux : Mux  Inputs=2
  socCellMux : Mux  Inputs=2
  socParallelAssemblyMux : Mux  Inputs=2
  temperatureCellMux : Mux  Inputs=2
  vCellMux : Mux  Inputs=2
  vParallelAssemblyMux : Mux  Inputs=2
  + : PMIOPort  Side=Left
  - : PMIOPort  Port=2  Side=Right
  AmbH : PMIOPort  Port=3  Side=Right  ConnectionType=Connection: foundation.thermal.thermal
  ClntH : PMIOPort  Port=4  Side=Right  ConnectionType=Connection: foundation.thermal.thermal
  iCell : Outport
  numCyclesCell : Outport  Port=2
  socCell : Outport  Port=3
  socParallelAssembly : Outport  Port=4
  temperatureCell : Outport  Port=5
  vCell : Outport  Port=6
  vParallelAssembly : Outport  Port=7
  wires:
  Module_1_outputs/1 -> [iCell1]
  iCellMux/1 -> iCell/1
  [iCell1] -> iCellMux/1
  Module_1_outputs/2 -> [numCyclesCell1]
  numCyclesCellMux/1 -> numCyclesCell/1
  [numCyclesCell1] -> numCyclesCellMux/1
  Module_1_outputs/3 -> [socCell1]
  socCellMux/1 -> socCell/1
  [socCell1] -> socCellMux/1
  Module_1_outputs/4 -> [socParallelAssembly1]
  socParallelAssemblyMux/1 -> socParallelAssembly/1
  [socParallelAssembly1] -> socParallelAssemblyMux/1
  Module_1_outputs/5 -> [temperatureCell1]
  temperatureCellMux/1 -> temperatureCell/1
  [temperatureCell1] -> temperatureCellMux/1
  Module_1_outputs/6 -> [vCell1]
  vCellMux/1 -> vCell/1
  [vCell1] -> vCellMux/1
  Module_1_outputs/7 -> [vParallelAssembly1]
  vParallelAssemblyMux/1 -> vParallelAssembly/1
  [vParallelAssembly1] -> vParallelAssemblyMux/1
  Module2_outputs/1 -> [iCell2]
  [iCell2] -> iCellMux/2
  Module2_outputs/2 -> [numCyclesCell2]
  [numCyclesCell2] -> numCyclesCellMux/2
  Module2_outputs/3 -> [socCell2]
  [socCell2] -> socCellMux/2
  Module2_outputs/4 -> [socParallelAssembly2]
  [socParallelAssembly2] -> socParallelAssemblyMux/2
  Module2_outputs/5 -> [temperatureCell2]
  [temperatureCell2] -> temperatureCellMux/2
  Module2_outputs/6 -> [vCell2]
  [vCell2] -> vCellMux/2
  Module2_outputs/7 -> [vParallelAssembly2]
  [vParallelAssembly2] -> vParallelAssemblyMux/2
  connections:
  Module_1/LConn3 -- Module2/LConn3 -- +/RConn1
  Module_1/RConn1 -- Module2/RConn1 -- -/RConn1
  AmbH_To_1/LConn1 -- Module_1/LConn2
  AmbH/RConn1 -- AmbH_From_1/LConn1 -- AmbH_From_2/LConn1
  AmbH_To_2/LConn1 -- Module2/LConn2
  ClntH_To_1/LConn1 -- Module_1/LConn1
  ClntH/RConn1 -- ClntH_From_1/LConn1 -- ClntH_From_2/LConn1
  ClntH_To_2/LConn1 -- Module2/LConn1
